simulink model "Model_2"  (R2020a)
settings: Solver=VariableStepAuto  StartTime=0.0  StopTime=10.0  RelTol=1e-3
libraries: dspsigops x3, dsparch4 x3
settings Model: Creator=User  LastModifiedBy=User

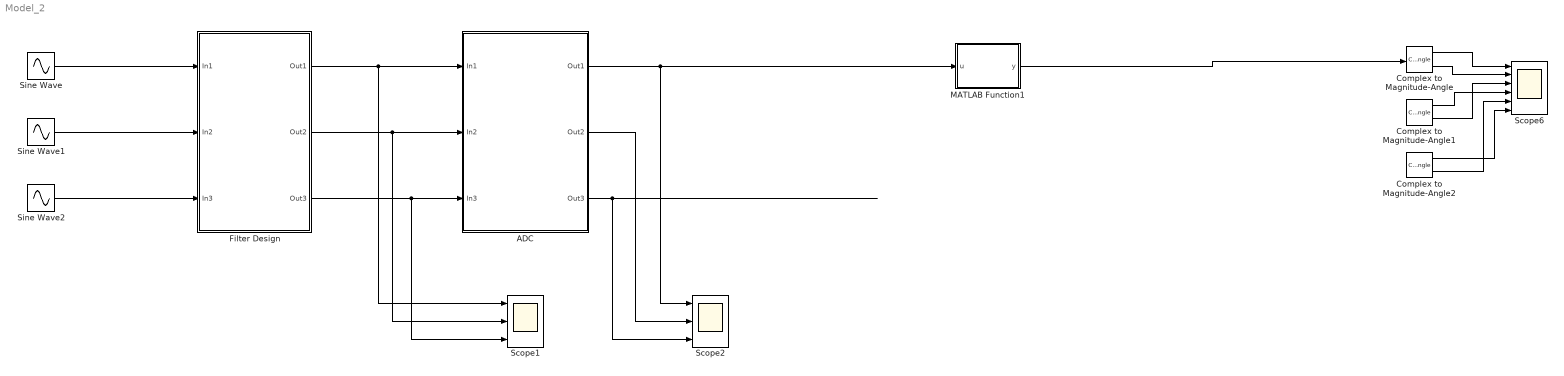
== system Model_2 ==
  ADC : Subsystem
  Complex to Magnitude-Angle : ComplexToMagnitudeAngle
  Complex to Magnitude-Angle1 : ComplexToMagnitudeAngle
  Complex to Magnitude-Angle2 : ComplexToMagnitudeAngle
  Filter Design : Subsystem
  MATLAB Function1 : MATLAB Function  TreatAsAtomicUnit=on
  Scope1 : Scope  NumInputPorts=3
  Scope2 : Scope  NumInputPorts=3
  Scope6 : Scope  NumInputPorts=6
  Sine Wave : Sin  Amplitude=20  Frequency=2*pi*(50)  SampleTime=0
  Sine Wave1 : Sin  Frequency=2*pi*50  SampleTime=0
  Sine Wave2 : Sin  Frequency=2*pi*50  Phase=-2*pi/3  SampleTime=0
  wires:
  Sine Wave/1 -> Filter Design/1(In1)
  Sine Wave1/1 -> Filter Design/2(In2)
  Filter Design/1(Out1) -> Scope1/1, ADC/1(In1)
  Sine Wave2/1 -> Filter Design/3(In3)
  Filter Design/2(Out2) -> Scope1/2, ADC/2(In2)
  Filter Design/3(Out3) -> Scope1/3, ADC/3(In3)
  ADC/2(Out2) -> Scope2/2
  ADC/3(Out3) -> Scope2/3
  Complex to Magnitude-Angle1/2 -> Scope6/3
  Complex to Magnitude-Angle2/2 -> Scope6/5
  Complex to Magnitude-Angle1/1 -> Scope6/4
  Complex to Magnitude-Angle2/1 -> Scope6/6
  ADC/1(Out1) -> MATLAB Function1/1(u), Scope2/1
  MATLAB Function1/1(y) -> Complex to Magnitude-Angle/1
  Complex to Magnitude-Angle/1 -> Scope6/1
  Complex to Magnitude-Angle/2 -> Scope6/2

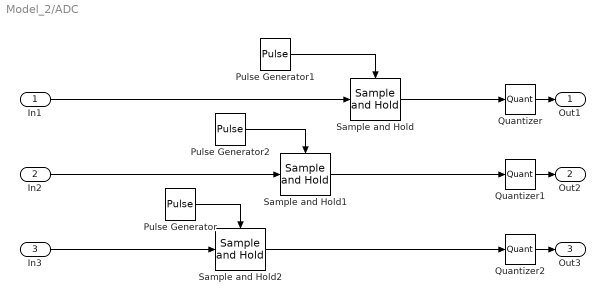
== system Model_2/ADC ==
  In1 : Inport
  In2 : Inport  Port=2
  In3 : Inport  Port=3
  Pulse Generator : DiscretePulseGenerator  PulseType=Time based  Period=0.001  PulseWidth=5
  Pulse Generator1 : DiscretePulseGenerator  PulseType=Time based  Period=0.001  PulseWidth=5
  Pulse Generator2 : DiscretePulseGenerator  PulseType=Time based  Period=0.001  PulseWidth=5
  Quantizer : Quantizer  QuantizationInterval=0.1
  Quantizer1 : Quantizer  QuantizationInterval=0.1
  Quantizer2 : Quantizer  QuantizationInterval=0.1
  Sample and Hold : dspsigops/Sample and Hold  trig=Rising edge  initCond=0  latchinput=off
  Sample and Hold1 : dspsigops/Sample and Hold  trig=Rising edge  initCond=0  latchinput=off
  Sample and Hold2 : dspsigops/Sample and Hold  trig=Rising edge  initCond=0  latchinput=off
  Out1 : Outport
  Out2 : Outport  Port=2
  Out3 : Outport  Port=3
  wires:
  In1/1 -> Sample and Hold/1
  Sample and Hold2/1 -> Quantizer2/1
  Sample and Hold1/1 -> Quantizer1/1
  Pulse Generator1/1 -> Sample and Hold/Trigger
  In2/1 -> Sample and Hold1/1
  Pulse Generator/1 -> Sample and Hold2/Trigger
  Quantizer2/1 -> Out3/1
  Sample and Hold/1 -> Quantizer/1
  Pulse Generator2/1 -> Sample and Hold1/Trigger
  Quantizer/1 -> Out1/1
  Quantizer1/1 -> Out2/1
  In3/1 -> Sample and Hold2/1

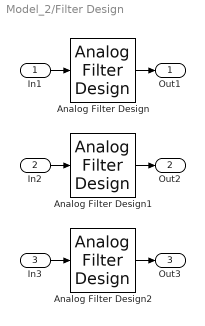
== system Model_2/Filter Design ==
  In1 : Inport
  In2 : Inport  Port=2
  In3 : Inport  Port=3
  Analog Filter Design : dsparch4/Analog Filter Design  method=Butterworth  filttype=Lowpass  N=8  Wlo=2*pi*60  Whi=80  Rp=2  Rs=40
  Analog Filter Design1 : dsparch4/Analog Filter Design  method=Butterworth  filttype=Lowpass  N=8  Wlo=2*pi*60  Whi=80  Rp=2  Rs=40
  Analog Filter Design2 : dsparch4/Analog Filter Design  method=Butterworth  filttype=Lowpass  N=8  Wlo=2*pi*60  Whi=80  Rp=2  Rs=40
  Out1 : Outport
  Out2 : Outport  Port=2
  Out3 : Outport  Port=3
  wires:
  In2/1 -> Analog Filter Design1/1
  Analog Filter Design1/1 -> Out2/1
  In1/1 -> Analog Filter Design/1
  Analog Filter Design2/1 -> Out3/1
  In3/1 -> Analog Filter Design2/1
  Analog Filter Design/1 -> Out1/1

== matlab function Model_2/MATLAB Function1 ==
  settings: updateMethod=CONTINUOUS
  data: u input; y output
function y = fcn(u)



t=0:0.001:0.02;
N = 20;
f0=50;
theta = 2*pi/N;
xt = u;

xn = zeros(1,N);

for Xn = [0:1:N-1]
    xn(Xn+1)=*cos(Xn*theta);
end


Xc = zeros(1,N);
for Xn = [0:1:N-1]
    Xc(Xn+1)=cos(Xn*theta);
end

N = 20;
theta = 2*pi/N;
Xs = zeros(1,N);
for Xn = [0:1:N-1]
    Xs(Xn+1)=sin(Xn*theta);
end


sum_c =0;
for Xn = [0:1:N-1]
    temp=xn(Xn+1)*Xc(Xn+1);
    sum_c=sum_c+temp;
end

Xc_N_1 = sqrt(2)/N*sum_c;

sum_s =0;
for Xn = [0:1:N-1]
    temp=xn(Xn+1)*Xs(Xn+1);
    sum_s=sum_s+temp;
end

Xs_N_1 = sqrt(2)/N*sum_s;

X_N_1 = Xc_N_1-j*Xs_N_1;
y = X_N_1;

y = X_N_1 ;
